simulink model "PartitionWallMatrixSim"  (R2018b)
settings: Solver=FixedStepAuto  StartTime=0.0  StopTime=1000000.0  FixedStep=5  RelTol=1e-3
values from neighbouring files (symbols this model uses):
  conductiveHconnectMatrix = [ ... (first row only)    [PartitionWallMatrix.m]
undefined symbols (not defined in the file or in its folder): DiscIntNeverNeededParam, roomVol
settings Model: Creator=cpp14rcj  LastModifiedBy=cpp14rcj

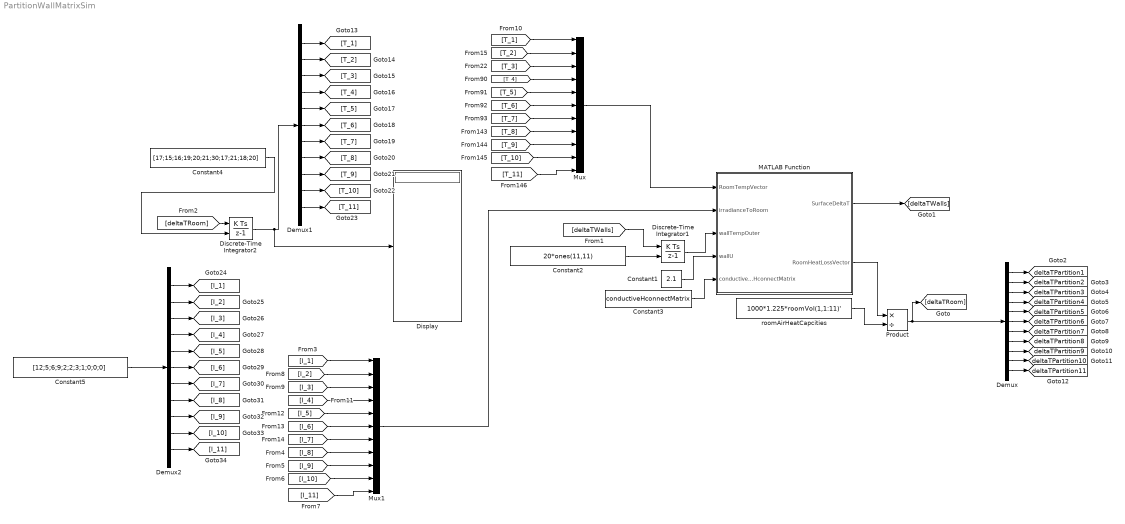
== system PartitionWallMatrixSim ==
  Constant1 : Constant  Value=2.1
  Constant2 : Constant  Value=20*ones(11,11)
  Constant3 : Constant  Value=conductiveHconnectMatrix
  Constant4 : Constant  Value=[17;15;16;19;20;21;30;17;21;18;20]
  Constant5 : Constant  Value=[12;5;6;9;2;2;3;1;0;0;0]
  Demux : Demux  Outputs=11
  Demux1 : Demux  Outputs=11
  Demux2 : Demux  Outputs=11
  Discrete-Time Integrator1 : DiscreteIntegrator  InitialConditionSource=external  SampleTime=-1  ICPrevOutput=DiscIntNeverNeededParam  ICPrevScaledInput=DiscIntNeverNeededParam
  Discrete-Time Integrator2 : DiscreteIntegrator  InitialConditionSource=external  SampleTime=-1  ICPrevOutput=DiscIntNeverNeededParam  ICPrevScaledInput=DiscIntNeverNeededParam
  Display : Display
  MATLAB Function : MATLAB Function  TreatAsAtomicUnit=on
  Mux : Mux  Inputs=11
  Mux1 : Mux  Inputs=11
  Product : Product  Inputs=*/
  roomAirHeatCapcities : Constant  Value=1000*1.225*roomVol(1,1:11)'
  tag scope: deltaTPartition10=global, deltaTPartition11=global, deltaTPartition1=global, deltaTPartition2=global, deltaTPartition3=global, deltaTPartition4=global, deltaTPartition5=global, deltaTPartition6=global, deltaTPartition7=global, deltaTPartition8=global, deltaTPartition9=global
  wires:
  Constant1/1 -> MATLAB Function/4(wallU)
  Discrete-Time Integrator1/1 -> MATLAB Function/3(wallTempOuter)
  Constant2/1 -> Discrete-Time Integrator1/2
  [deltaTWalls] -> Discrete-Time Integrator1/1
  Constant3/1 -> MATLAB Function/5(conductiveHconnectMatrix)
  MATLAB Function/2(RoomHeatLossVector) -> Product/1
  MATLAB Function/1(SurfaceDeltaT) -> [deltaTWalls]
  roomAirHeatCapcities/1 -> Product/2
  Product/1 -> [deltaTRoom], Demux/1
  Demux/1 -> [deltaTPartition1]
  [T_1] -> Mux/1
  [T_2] -> Mux/2
  [T_3] -> Mux/3
  [T_4] -> Mux/4
  [T_5] -> Mux/5
  [T_6] -> Mux/6
  [T_7] -> Mux/7
  [T_8] -> Mux/8
  [T_9] -> Mux/9
  [T_10] -> Mux/10
  [T_11] -> Mux/11
  Mux/1 -> MATLAB Function/1(RoomTempVector)
  Demux/2 -> [deltaTPartition2]
  Demux/4 -> [deltaTPartition4]
  Demux/5 -> [deltaTPartition5]
  Demux/6 -> [deltaTPartition6]
  Demux/7 -> [deltaTPartition7]
  Demux/8 -> [deltaTPartition8]
  Demux/9 -> [deltaTPartition9]
  Demux/11 -> [deltaTPartition11]
  Demux/10 -> [deltaTPartition10]
  Demux/3 -> [deltaTPartition3]
  Demux1/1 -> [T_1]
  Demux1/2 -> [T_2]
  Demux1/3 -> [T_3]
  Demux1/4 -> [T_4]
  Demux1/5 -> [T_5]
  Demux1/6 -> [T_6]
  Demux1/7 -> [T_7]
  Demux1/8 -> [T_8]
  Demux1/9 -> [T_9]
  Demux1/10 -> [T_10]
  Demux1/11 -> [T_11]
  Constant4/1 -> Discrete-Time Integrator2/2
  [deltaTRoom] -> Discrete-Time Integrator2/1
  Discrete-Time Integrator2/1 -> Display/1, Demux1/1
  [I_8] -> Mux1/8
  [I_1] -> Mux1/1
  Mux1/1 -> MATLAB Function/2(irradianceToRoom)
  [I_2] -> Mux1/2
  [I_3] -> Mux1/3
  [I_10] -> Mux1/10
  [I_7] -> Mux1/7
  [I_5] -> Mux1/5
  [I_4] -> Mux1/4
  [I_11] -> Mux1/11
  [I_9] -> Mux1/9
  [I_6] -> Mux1/6
  Demux2/8 -> [I_8]
  Demux2/7 -> [I_7]
  Demux2/5 -> [I_5]
  Demux2/3 -> [I_3]
  Demux2/1 -> [I_1]
  Demux2/10 -> [I_10]
  Demux2/4 -> [I_4]
  Demux2/11 -> [I_11]
  Demux2/2 -> [I_2]
  Demux2/6 -> [I_6]
  Demux2/9 -> [I_9]
  Constant5/1 -> Demux2/1

== matlab function PartitionWallMatrixSim/MATLAB Function ==
  data: RoomTempVector input; irradianceToRoom input; SurfaceDeltaT output; wallTempOuter input; wallU input; conductiveHconnectMatrix input; RoomHeatLossVector output
function [SurfaceDeltaT,RoomHeatLossVector] = fcn(RoomTempVector,irradianceToRoom,wallTempOuter,wallU,conductiveHconnectMatrix)


TempRoomRow=repmat(RoomTempVector,1,11);

SurfaceHeatCapPerM2=(0.0155*1*1)*800*1090; %plaster specs thickness=(0.0125m plasterboard+0.003m skim), 1090 j/k/kg, 800kg/m3

convectiveToSurface=(2.4*conductiveHconnectMatrix)*5.1.*(TempRoomRow-wallTempOuter);

conductiveToOppositeSurface=(2.4*conductiveHconnectMatrix)*(wallU*2).*(wallTempOuter-wallTempOuter');
convectiveToSurface(isnan(convectiveToSurface))=0;
conductiveToOppositeSurface(isnan(conductiveToOppositeSurface))=0;

fractionalArea=conductiveHconnectMatrix./repmat(sum(conductiveHconnectMatrix,2),1,11);
radiativeToSurface=fractionalArea.*repmat(irradianceToRoom,1,11);


SurfaceHeatChange=(convectiveToSurface-conductiveToOppositeSurface)+radiativeToSurface;


SurfaceDeltaT=SurfaceHeatChange./(SurfaceHeatCapPerM2*2.4*conductiveHconnectMatrix);
SurfaceDeltaT(isnan(SurfaceDeltaT))=0;
RoomHeatLossVector=-sum(convectiveToSurface,2);
